simulink model "GFL_hw"  (R2023b)
settings: Solver=FixedStepAuto  StartTime=0.0  StopTime=Inf  RelTol=1e-3  EnableMultiTasking=on
values from neighbouring files (symbols this model uses):
  alpha_c = 2*pi*400    (= 2513.27412287)    [init_hw.m]    (also in init_psc_hw.m)
  L_f = 1e-3    (= 0.001)    [init_hw.m]    (also in init_psc_hw.m)
  T_pwm = f_clk/(div*f_sw*carr)    (= 9000)    [init_hw.m]    (also in init_psc_hw.m)
  T_s = 1/(2*f_sw)    (= 0.0001)    [init_hw.m]    (also in init_psc_hw.m)
  u_gN = 24    [init_hw.m]    (also in init_psc_hw.m)
  w0_pll = 2*pi*20    (= 125.663706144)    [init_hw.m]    (also in init_psc_hw.m)
undefined symbols (not defined in the file or in its folder): Down, GPTRIP1SEL, GPTRIP2SEL, TZ1, TZ2, Up, w_g
libraries: c2802xlib x14, c2806xlib x5
settings Model: SimulationMode=external  ExtModeTrigDuration=15  Creator=maatt  LastModifiedBy=maatt
settings OptimizationCC: DefaultUnderspecifiedDataType=single  EnhancedBackFolding=on  PassReuseOutputArgsAs=Individual arguments  MaxStackSize=1024  OptimizeBlockOrder=speed  DifferentSizesBufferReuse=on  OptimizationCustomize=off  EfficientTunableParamExpr=on
settings DebuggingCC: ParameterTunabilityLossMsg=error
settings HardwareCC: ProdBitPerChar=16  ProdBitPerInt=16  ProdBitPerPointer=32  ProdBitPerSizeT=32  ProdBitPerPtrDiffT=32  ProdLargestAtomicInteger=Integer  ProdLargestAtomicFloat=None  ProdWordSize=16  ProdLongLongMode=on  ProdHWDeviceType=Texas Instruments->C2000  HardwareBoardFeatureSet=SoCBlockset
settings ModelReferenceCC: ModelReferenceNumInstancesAllowed=Single
settings SFSimCC: MATLABDynamicMemAlloc=off
settings RTWCC: Description=Embedded Coder  SystemTargetFile=ert.tlc  HardwareBoard=TI Piccolo F28069M LaunchPad  TemplateMakefile=ert_default_tmf  Toolchain=Texas Instruments Code Composer Studio (C2000)  CodeProfilingSaveOptions=MetricsOnly
settings CodeAppCC: ForceParamTrailComments=on  IgnoreCustomStorageClasses=off  OperatorAnnotations=on  SimulinkDataObjDesc=on  SFDataObjDesc=on  InsertBlockDesc=on
settings ERTTargetCC: CodeReplacementLibrary=TI C28x  ExtModeTransport=4  ExtModeStaticAlloc=on  ExtModeAutomaticAllocSize=off  ExtModeStaticAllocSize=2000  ExtModeMexFile=ext_xcp  ExtModeIntrfLevel=Level2 - Open

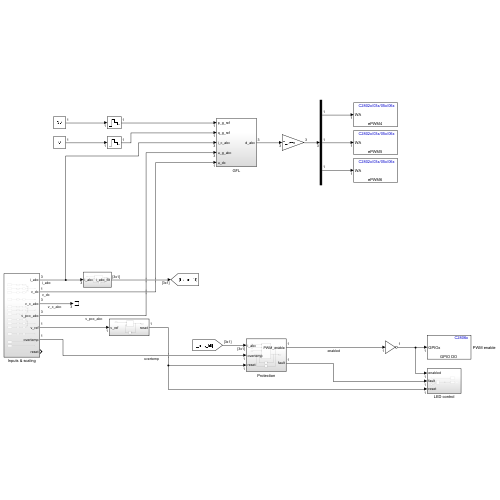
[thumbnail: Simulink's stored preview of the top-level diagram]
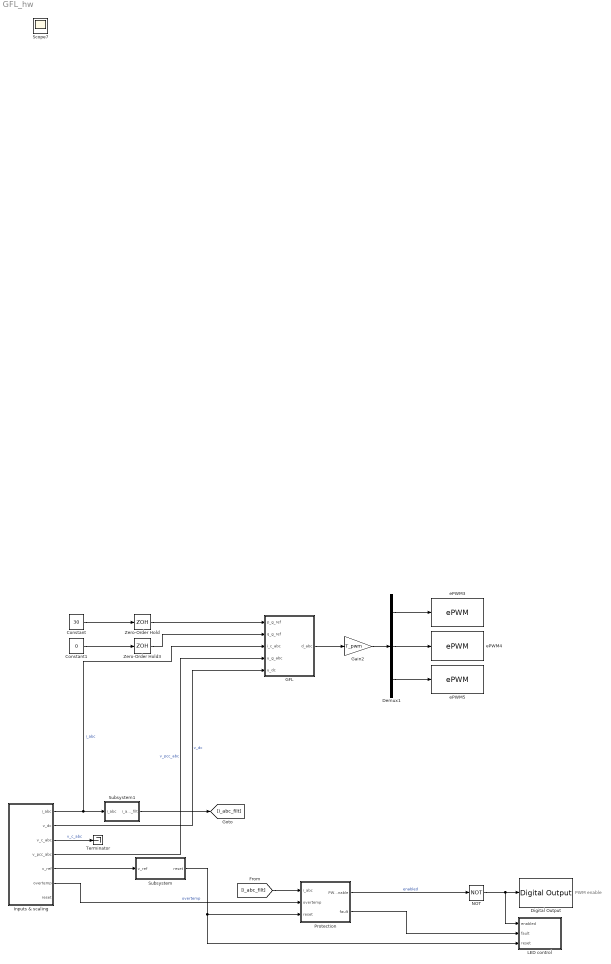
== system GFL_hw ==
  note: PWM enable
  Constant : Constant  Value=30  SampleTime=T_s
  Constant1 : Constant  Value=0  SampleTime=T_s
  Demux1 : Demux  Outputs=3
  Digital Output : c2806xlib/Digital Output  GPIO_Number=GPIO50~GPIO55  GPIO_Bit0=off  GPIO_BIT0_Toggle=off  GPIO_Bit1=off  GPIO_BIT1_Toggle=off  GPIO_Bit2=off  GPIO_BIT2_Toggle=off  GPIO_Bit3=off  GPIO_BIT3_Toggle=off  GPIO_Bit4=on  GPIO_BIT4_Toggle=off  GPIO_Bit5=off  GPIO_BIT5_Toggle=off  GPIO_Bit6=off  GPIO_BIT6_Toggle=off  GPIO_Bit7=off  GPIO_BIT7_Toggle=off
  GFL : Subsystem
  Gain2 : Gain  Gain=T_pwm
  Inputs & scaling : Subsystem
  LED control : Subsystem
  NOT : Logic  Operator=NOT  IconShape=distinctive  AllPortsSameDT=off  OutDataTypeStr=boolean
  Protection : Subsystem
  Subsystem : Subsystem
  Subsystem1 : Subsystem
  Terminator : Terminator
  Zero-Order Hold : ZeroOrderHold  SampleTime=T_s
  Zero-Order Hold3 : ZeroOrderHold  SampleTime=T_s
  ePWM3 : c2802xlib/ePWM  PwmType=C2000  useModule=ePWM4  ePWMxLINKTBPRD=Not Linked  periodUnits=Clock cycles  timerSource=Specify via dialog  timerPeriod_clk=T_pwm + 1  timerPeriod_sec=0.0001  tbshadow=Counter equals to zero  countingMode=Up-Down  phaseActiveEnable=Disable  phaseDirection=Count down after sync  phaseActive=0  synchronizationEnable=off  dcaevt1Sync=off  dcbevt1Sync=off  synchronizationOption=Counter equals to zero (CTR=Zero)  dcbevt1SyncOut=off  dcaevt1SyncOut=off  cmpdSyncOut=off  cmpcSyncOut=off  cmpbSyncOut=off  zeroSyncOut=off  swfSyncOut=off  perSynchronizationOption=Counter equals to period (CTR=PRD)  clockPrescale=1  HSclockPrescale=1  enswap=off  ePWMxAStatus=on  ePWMxAactionLogic1=Do nothing  ePWMxAactionLogic2=Do nothing  ePWMxAactionLogic3=Clear  ePWMxAactionLogic4=Set  ePWMxAactionLogic5=Do nothing  ePWMxAactionLogic6=Do nothing  ePWMxACSFenable=off  ePWMxACSFvalue=Forcing disable  ePWMxASFreload=Zero  ePWMxBStatus=off  ePWMxBactionLogic1=Set  ePWMxBactionLogic2=Clear  ePWMxBactionLogic3=Do nothing  ePWMxBactionLogic4=Do nothing  ePWMxBactionLogic5=Clear  ePWMxBactionLogic6=Set  ePWMxBCSFenable=off  ePWMxBCSFvalue=Forcing disable  ePWMxBSFreload=Zero  ePWNxBOutWay=on  ePWMxLINKCMPA=Not Linked  CMPAUnits=Clock cycles  CMPASource=Input port  CMPAValue_per=50  CMPAValue_clk=T_pwm/2  enCMPAshadow=Counter equals to zero (CTR=Zero)  ePWMxLINKCMPB=Not Linked  CMPBUnits=Clock cycles  CMPBSource=Specify via dialog  CMPBValue_per=50  CMPBValue_clk=T_pwm/2  enCMPBshadow=Counter equals to zero (CTR=Zero)  ePWMxLINKCMPC=Not Linked  CMPCUnits=Clock cycles  CMPCSource=Specify via dialog  CMPCValue_per=50  CMPCValue_clk=32000  enCMPCshadow=Counter equals to zero (CTR=Zero)  ePWMxLINKCMPD=Not Linked  CMPDUnits=Clock cycles  CMPDSource=Specify via dialog  CMPDValue_per=50  CMPDValue_clk=32000  enCMPDshadow=Counter equals to zero (CTR=Zero)  enableDBePWMxA=on  enableDBePWMxB=on  enhalfcycle=off  DBpolarity=Active high complementary (AHC)  DBedgeDelay=Positive  DBSource_ePWMxA=ePWMxA  DBSource_ePWMxB=ePWMxA  DBPeriodUnits=Clock cycles  DBperiodSource=Specify via dialog  REDperiod=15  FEDperiod=15  REDperiod_sec=0  FEDperiod_sec=0  LoadModeDBRED=Immediate without using shadow  LoadModeDBFED=Immediate without using shadow  adcstartModuleA=off  adcrequestEventA=First event  adcstartEventA=Counter equals to zero (CTR=Zero)  adcstartEventA_type2=Digital Compare Module A Event 1 start of conversion (DCAEVT1.soc)  adcstartModuleB=off  adcrequestEventB=First event  adcstartEventB=Counter equals to zero (CTR=Zero)  adcstartEventB_type2=Counter equals to zero (CTR=Zero)  intEn=off  intPrd=First event  intSel=Counter equals to zero (CTR=Zero)  intSel_type2=Counter equals to zero (CTR=Zero)  hrpe=off  enHRPWM=off  HRPWM_LoadMode=Counter equals to period (CTR=PRD)  HRPWM_CTLMode=Duty or Period control mode  HRPWM_EDGMode=Both edge  hrpeb=off  enHRPWMB=off  HRPWM_LoadModeB=Counter equals to zero (CTR=ZERO)  HRPWM_CTLModeB=Duty or Period control mode  HRPWM_EDGModeB=Both edge  enHRDBRED=off  enHRDBFED=off  enSFO=on  enautoconv=on  chopperEnable=off  chopperFrequency=1  chopperFirstwidth=1  chopperDuty=12.5%  tripZonesource=Specify via dialog  tzselOSHT1=off  tzselOSHT2=off  tzselOSHT3=off  tzselOSHDCAEV1=off  tzselOSHDCBEV1=off  tzselCBC1=off  tzselCBC2=off  tzselCBC3=off  tzselCBCDCAEV2=off  tzselCBCDCBEV2=off  tzselOSHT4=off  tzselOSHT5=off  tzselOSHT6=off  tzselCBC4=off  tzselCBC5=off  tzselCBC6=off  enTzOstIntr=off  enTzCbcIntr=off  enTzDCAEVT1Intr=off  enTzDCAEVT2Intr=off  enTzDCBEVT1Intr=off  enTzDCBEVT2Intr=off  ePWMxAforced=No action  ePWMxBforced=No action  DCAEVT1forced=No action  DCBEVT1forced=No action  DCAEVT2forced=No action  DCBEVT2forced=No action  dcah=Trip Zone 1 input (TZ1)  dcal=Trip Zone 1 input (TZ1)  dcbh=Trip Zone 1 input (TZ1)  dcbl=Trip Zone 1 input (TZ1)  dcah_type2=GPTRIP1SEL/(TZ1)  dcal_type2=GPTRIP2SEL/(TZ2)  dcbh_type2=GPTRIP1SEL/(TZ1)  dcbl_type2=GPTRIP2SEL/(TZ2)  gendcaevt1=Event disabled  gendcaevt2=Event disabled  gendcbevt1=Event disabled  gendcbevt2=Event disabled  dcaevt1src=DCAEVT1 with sync  dcaevt2src=DCAEVT2 with sync  dcbevt1src=DCBEVT1 with sync  dcbevt2src=DCBEVT2 with sync  pulsesel=Counter equals to zero (CTR=Zero)  blankinv=off  blankoffset=0  blankwidth=0  evsrcsel=Filtered version of DCAEVT1 (DCAEVT1FILT)  encape=off
      settings: LibrarySourceBlock=c2806xlib/ePWM
  ePWM4 : c2802xlib/ePWM  PwmType=C2000  useModule=ePWM5  ePWMxLINKTBPRD=Not Linked  periodUnits=Clock cycles  timerSource=Specify via dialog  timerPeriod_clk=T_pwm + 1  timerPeriod_sec=0.0001  tbshadow=Counter equals to zero  countingMode=Up-Down  phaseActiveEnable=Disable  phaseDirection=Count down after sync  phaseActive=0  synchronizationEnable=off  dcaevt1Sync=off  dcbevt1Sync=off  synchronizationOption=Counter equals to zero (CTR=Zero)  dcbevt1SyncOut=off  dcaevt1SyncOut=off  cmpdSyncOut=off  cmpcSyncOut=off  cmpbSyncOut=off  zeroSyncOut=off  swfSyncOut=off  perSynchronizationOption=Counter equals to period (CTR=PRD)  clockPrescale=1  HSclockPrescale=1  enswap=off  ePWMxAStatus=on  ePWMxAactionLogic1=Do nothing  ePWMxAactionLogic2=Do nothing  ePWMxAactionLogic3=Clear  ePWMxAactionLogic4=Set  ePWMxAactionLogic5=Do nothing  ePWMxAactionLogic6=Do nothing  ePWMxACSFenable=off  ePWMxACSFvalue=Forcing disable  ePWMxASFreload=Zero  ePWMxBStatus=off  ePWMxBactionLogic1=Set  ePWMxBactionLogic2=Clear  ePWMxBactionLogic3=Do nothing  ePWMxBactionLogic4=Do nothing  ePWMxBactionLogic5=Clear  ePWMxBactionLogic6=Set  ePWMxBCSFenable=off  ePWMxBCSFvalue=Forcing disable  ePWMxBSFreload=Zero  ePWNxBOutWay=on  ePWMxLINKCMPA=Not Linked  CMPAUnits=Clock cycles  CMPASource=Input port  CMPAValue_per=50  CMPAValue_clk=T_pwm/2  enCMPAshadow=Counter equals to zero (CTR=Zero)  ePWMxLINKCMPB=Not Linked  CMPBUnits=Clock cycles  CMPBSource=Specify via dialog  CMPBValue_per=50  CMPBValue_clk=T_pwm/2  enCMPBshadow=Counter equals to zero (CTR=Zero)  ePWMxLINKCMPC=Not Linked  CMPCUnits=Clock cycles  CMPCSource=Specify via dialog  CMPCValue_per=50  CMPCValue_clk=32000  enCMPCshadow=Counter equals to zero (CTR=Zero)  ePWMxLINKCMPD=Not Linked  CMPDUnits=Clock cycles  CMPDSource=Specify via dialog  CMPDValue_per=50  CMPDValue_clk=32000  enCMPDshadow=Counter equals to zero (CTR=Zero)  enableDBePWMxA=on  enableDBePWMxB=on  enhalfcycle=off  DBpolarity=Active high complementary (AHC)  DBedgeDelay=Positive  DBSource_ePWMxA=ePWMxA  DBSource_ePWMxB=ePWMxA  DBPeriodUnits=Clock cycles  DBperiodSource=Specify via dialog  REDperiod=15  FEDperiod=15  REDperiod_sec=0  FEDperiod_sec=0  LoadModeDBRED=Immediate without using shadow  LoadModeDBFED=Immediate without using shadow  adcstartModuleA=off  adcrequestEventA=First event  adcstartEventA=Counter equals to zero (CTR=Zero)  adcstartEventA_type2=Digital Compare Module A Event 1 start of conversion (DCAEVT1.soc)  adcstartModuleB=off  adcrequestEventB=First event  adcstartEventB=Counter equals to zero (CTR=Zero)  adcstartEventB_type2=Counter equals to zero (CTR=Zero)  intEn=off  intPrd=First event  intSel=Counter equals to zero (CTR=Zero)  intSel_type2=Counter equals to zero (CTR=Zero)  hrpe=off  enHRPWM=off  HRPWM_LoadMode=Counter equals to period (CTR=PRD)  HRPWM_CTLMode=Duty or Period control mode  HRPWM_EDGMode=Both edge  hrpeb=off  enHRPWMB=off  HRPWM_LoadModeB=Counter equals to zero (CTR=ZERO)  HRPWM_CTLModeB=Duty or Period control mode  HRPWM_EDGModeB=Both edge  enHRDBRED=off  enHRDBFED=off  enSFO=on  enautoconv=on  chopperEnable=off  chopperFrequency=1  chopperFirstwidth=1  chopperDuty=12.5%  tripZonesource=Specify via dialog  tzselOSHT1=off  tzselOSHT2=off  tzselOSHT3=off  tzselOSHDCAEV1=off  tzselOSHDCBEV1=off  tzselCBC1=off  tzselCBC2=off  tzselCBC3=off  tzselCBCDCAEV2=off  tzselCBCDCBEV2=off  tzselOSHT4=off  tzselOSHT5=off  tzselOSHT6=off  tzselCBC4=off  tzselCBC5=off  tzselCBC6=off  enTzOstIntr=off  enTzCbcIntr=off  enTzDCAEVT1Intr=off  enTzDCAEVT2Intr=off  enTzDCBEVT1Intr=off  enTzDCBEVT2Intr=off  ePWMxAforced=No action  ePWMxBforced=No action  DCAEVT1forced=No action  DCBEVT1forced=No action  DCAEVT2forced=No action  DCBEVT2forced=No action  dcah=Trip Zone 1 input (TZ1)  dcal=Trip Zone 1 input (TZ1)  dcbh=Trip Zone 1 input (TZ1)  dcbl=Trip Zone 1 input (TZ1)  dcah_type2=GPTRIP1SEL/(TZ1)  dcal_type2=GPTRIP2SEL/(TZ2)  dcbh_type2=GPTRIP1SEL/(TZ1)  dcbl_type2=GPTRIP2SEL/(TZ2)  gendcaevt1=Event disabled  gendcaevt2=Event disabled  gendcbevt1=Event disabled  gendcbevt2=Event disabled  dcaevt1src=DCAEVT1 with sync  dcaevt2src=DCAEVT2 with sync  dcbevt1src=DCBEVT1 with sync  dcbevt2src=DCBEVT2 with sync  pulsesel=Counter equals to zero (CTR=Zero)  blankinv=off  blankoffset=0  blankwidth=0  evsrcsel=Filtered version of DCAEVT1 (DCAEVT1FILT)  encape=off
      settings: LibrarySourceBlock=c2806xlib/ePWM
  ePWM5 : c2802xlib/ePWM  PwmType=C2000  useModule=ePWM6  ePWMxLINKTBPRD=Not Linked  periodUnits=Clock cycles  timerSource=Specify via dialog  timerPeriod_clk=T_pwm + 1  timerPeriod_sec=0.0001  tbshadow=Counter equals to zero  countingMode=Up-Down  phaseActiveEnable=Disable  phaseDirection=Count down after sync  phaseActive=0  synchronizationEnable=off  dcaevt1Sync=off  dcbevt1Sync=off  synchronizationOption=Counter equals to zero (CTR=Zero)  dcbevt1SyncOut=off  dcaevt1SyncOut=off  cmpdSyncOut=off  cmpcSyncOut=off  cmpbSyncOut=off  zeroSyncOut=off  swfSyncOut=off  perSynchronizationOption=Counter equals to period (CTR=PRD)  clockPrescale=1  HSclockPrescale=1  enswap=off  ePWMxAStatus=on  ePWMxAactionLogic1=Do nothing  ePWMxAactionLogic2=Do nothing  ePWMxAactionLogic3=Clear  ePWMxAactionLogic4=Set  ePWMxAactionLogic5=Do nothing  ePWMxAactionLogic6=Do nothing  ePWMxACSFenable=off  ePWMxACSFvalue=Forcing disable  ePWMxASFreload=Zero  ePWMxBStatus=off  ePWMxBactionLogic1=Set  ePWMxBactionLogic2=Clear  ePWMxBactionLogic3=Do nothing  ePWMxBactionLogic4=Do nothing  ePWMxBactionLogic5=Clear  ePWMxBactionLogic6=Set  ePWMxBCSFenable=off  ePWMxBCSFvalue=Forcing disable  ePWMxBSFreload=Zero  ePWNxBOutWay=on  ePWMxLINKCMPA=Not Linked  CMPAUnits=Clock cycles  CMPASource=Input port  CMPAValue_per=50  CMPAValue_clk=T_pwm/2  enCMPAshadow=Counter equals to zero (CTR=Zero)  ePWMxLINKCMPB=Not Linked  CMPBUnits=Clock cycles  CMPBSource=Specify via dialog  CMPBValue_per=50  CMPBValue_clk=T_pwm/2  enCMPBshadow=Counter equals to zero (CTR=Zero)  ePWMxLINKCMPC=Not Linked  CMPCUnits=Clock cycles  CMPCSource=Specify via dialog  CMPCValue_per=50  CMPCValue_clk=32000  enCMPCshadow=Counter equals to zero (CTR=Zero)  ePWMxLINKCMPD=Not Linked  CMPDUnits=Clock cycles  CMPDSource=Specify via dialog  CMPDValue_per=50  CMPDValue_clk=32000  enCMPDshadow=Counter equals to zero (CTR=Zero)  enableDBePWMxA=on  enableDBePWMxB=on  enhalfcycle=off  DBpolarity=Active high complementary (AHC)  DBedgeDelay=Positive  DBSource_ePWMxA=ePWMxA  DBSource_ePWMxB=ePWMxA  DBPeriodUnits=Clock cycles  DBperiodSource=Specify via dialog  REDperiod=15  FEDperiod=15  REDperiod_sec=0  FEDperiod_sec=0  LoadModeDBRED=Immediate without using shadow  LoadModeDBFED=Immediate without using shadow  adcstartModuleA=off  adcrequestEventA=First event  adcstartEventA=Counter equals to zero (CTR=Zero)  adcstartEventA_type2=Digital Compare Module A Event 1 start of conversion (DCAEVT1.soc)  adcstartModuleB=off  adcrequestEventB=First event  adcstartEventB=Counter equals to zero (CTR=Zero)  adcstartEventB_type2=Counter equals to zero (CTR=Zero)  intEn=off  intPrd=First event  intSel=Counter equals to zero (CTR=Zero)  intSel_type2=Counter equals to zero (CTR=Zero)  hrpe=off  enHRPWM=off  HRPWM_LoadMode=Counter equals to period (CTR=PRD)  HRPWM_CTLMode=Duty or Period control mode  HRPWM_EDGMode=Both edge  hrpeb=off  enHRPWMB=off  HRPWM_LoadModeB=Counter equals to zero (CTR=ZERO)  HRPWM_CTLModeB=Duty or Period control mode  HRPWM_EDGModeB=Both edge  enHRDBRED=off  enHRDBFED=off  enSFO=on  enautoconv=on  chopperEnable=off  chopperFrequency=1  chopperFirstwidth=1  chopperDuty=12.5%  tripZonesource=Specify via dialog  tzselOSHT1=off  tzselOSHT2=off  tzselOSHT3=off  tzselOSHDCAEV1=off  tzselOSHDCBEV1=off  tzselCBC1=off  tzselCBC2=off  tzselCBC3=off  tzselCBCDCAEV2=off  tzselCBCDCBEV2=off  tzselOSHT4=off  tzselOSHT5=off  tzselOSHT6=off  tzselCBC4=off  tzselCBC5=off  tzselCBC6=off  enTzOstIntr=off  enTzCbcIntr=off  enTzDCAEVT1Intr=off  enTzDCAEVT2Intr=off  enTzDCBEVT1Intr=off  enTzDCBEVT2Intr=off  ePWMxAforced=No action  ePWMxBforced=No action  DCAEVT1forced=No action  DCBEVT1forced=No action  DCAEVT2forced=No action  DCBEVT2forced=No action  dcah=Trip Zone 1 input (TZ1)  dcal=Trip Zone 1 input (TZ1)  dcbh=Trip Zone 1 input (TZ1)  dcbl=Trip Zone 1 input (TZ1)  dcah_type2=GPTRIP1SEL/(TZ1)  dcal_type2=GPTRIP2SEL/(TZ2)  dcbh_type2=GPTRIP1SEL/(TZ1)  dcbl_type2=GPTRIP2SEL/(TZ2)  gendcaevt1=Event disabled  gendcaevt2=Event disabled  gendcbevt1=Event disabled  gendcbevt2=Event disabled  dcaevt1src=DCAEVT1 with sync  dcaevt2src=DCAEVT2 with sync  dcbevt1src=DCBEVT1 with sync  dcbevt2src=DCBEVT2 with sync  pulsesel=Counter equals to zero (CTR=Zero)  blankinv=off  blankoffset=0  blankwidth=0  evsrcsel=Filtered version of DCAEVT1 (DCAEVT1FILT)  encape=off
      settings: LibrarySourceBlock=c2806xlib/ePWM
  Scope7 : Scope
  wires:
  Demux1/1 -> ePWM3/1
  Demux1/2 -> ePWM4/1
  Gain2/1 -> Demux1/1
  Demux1/3 -> ePWM5/1
  [i_abc_filt] -> Protection/1(i_abc)
  Protection/1(PWM_enable) -> NOT/1  "enabled"
  Protection/2(fault) -> LED control/2(fault)
  Inputs & scaling/6(overtemp) -> Protection/2(overtemp)  "overtemp"
  Inputs & scaling/1(i_abc) -> GFL/3(i_c_abc), Subsystem1/1(i_abc)  "i_abc"
  Inputs & scaling/5(v_ref) -> Subsystem/1(v_ref)
  Inputs & scaling/3(v_c_abc) -> Terminator/1  "v_c_abc"
  Inputs & scaling/4(v_pcc_abc) -> GFL/4(u_g_abc)  "v_pcc_abc"
  NOT/1 -> LED control/1(enabled), Digital Output/1
  Subsystem/1(reset) -> Protection/3(reset), LED control/3(reset)
  Subsystem1/1(i_abc_filt) -> [i_abc_filt]
  GFL/1(d_abc) -> Gain2/1
  Zero-Order Hold/1 -> GFL/1(p_g_ref)
  Constant1/1 -> Zero-Order Hold3/1
  Zero-Order Hold3/1 -> GFL/2(q_g_ref)
  Inputs & scaling/2(v_dc) -> GFL/5(u_dc)  "v_dc"
  Constant/1 -> Zero-Order Hold/1

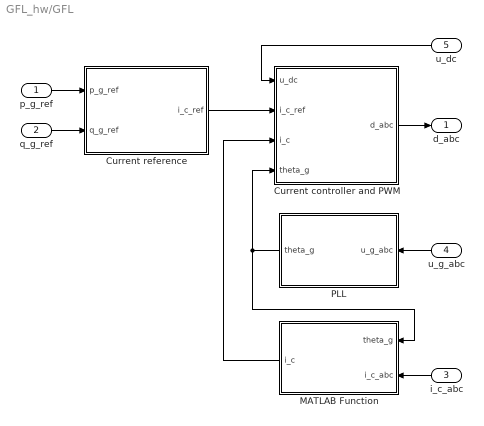
== system GFL_hw/GFL ==
  p_g_ref : Inport
  q_g_ref : Inport  Port=2
  i_c_abc : Inport  Port=3
  u_g_abc : Inport  Port=4
  u_dc : Inport  Port=5
  Current controller and PWM : Subsystem
  Current reference : MATLAB Function  TreatAsAtomicUnit=on
  MATLAB Function : MATLAB Function  TreatAsAtomicUnit=on
  PLL : Subsystem
  d_abc : Outport
  wires:
  i_c_abc/1 -> MATLAB Function/2(i_c_abc)
  Current controller and PWM/1(d_abc) -> d_abc/1
  Current reference/1(i_c_ref) -> Current controller and PWM/2(i_c_ref)
  MATLAB Function/1(i_c) -> Current controller and PWM/3(i_c)
  q_g_ref/1 -> Current reference/2(q_g_ref)
  p_g_ref/1 -> Current reference/1(p_g_ref)
  u_g_abc/1 -> PLL/1(u_g_abc)
  PLL/1(theta_g) -> MATLAB Function/1(theta_g), Current controller and PWM/4(theta_g)
  u_dc/1 -> Current controller and PWM/1(u_dc)

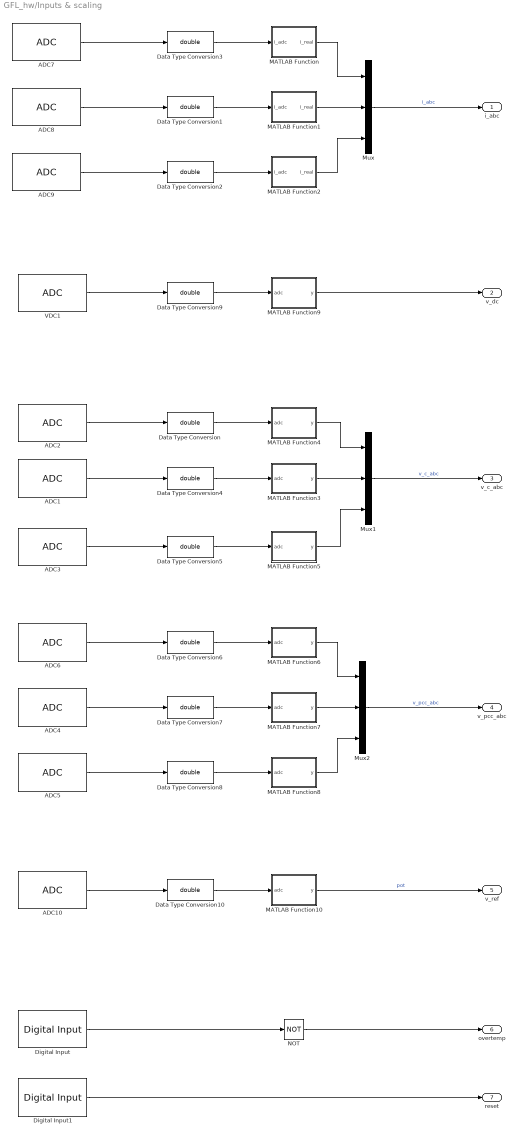
== system GFL_hw/Inputs & scaling ==
  ADC1 : c2802xlib/ADC  blkParamProc=C2000  ADCModule=1  samplingMode=Single sample mode  ADCResolution=12-bit (Single-ended input)  useSOC1=SOC5  useSOC2=SOC0_SOC1  SOCAcquisitionWindow=15  SOCTriggerSource=Software  SOCInterruptTrigger=No ADCINT  Ts=T_s  dType=uint16  postInterrupt=off  interruptSel=ADCINT1  ADCINTContinuous=off  endma=off  chdma=1  conv1=ADCINA5  conv2=ADCINA0 and ADCINB0  conv1_Type4=ADCIN0  conv2_Type4=ADCIN0 and ADCIN1
      settings: LibrarySourceBlock=c2806xlib/ADC
  ADC10 : c2802xlib/ADC  blkParamProc=C2000  ADCModule=1  samplingMode=Single sample mode  ADCResolution=12-bit (Single-ended input)  useSOC1=SOC10  useSOC2=SOC0_SOC1  SOCAcquisitionWindow=15  SOCTriggerSource=Software  SOCInterruptTrigger=No ADCINT  Ts=T_s  dType=uint16  postInterrupt=off  interruptSel=ADCINT1  ADCINTContinuous=off  endma=off  chdma=1  conv1=ADCINB2  conv2=ADCINA0 and ADCINB0  conv1_Type4=ADCIN0  conv2_Type4=ADCIN0 and ADCIN1
      settings: LibrarySourceBlock=c2806xlib/ADC
  ADC2 : c2802xlib/ADC  blkParamProc=C2000  ADCModule=1  samplingMode=Single sample mode  ADCResolution=12-bit (Single-ended input)  useSOC1=SOC4  useSOC2=SOC0_SOC1  SOCAcquisitionWindow=15  SOCTriggerSource=Software  SOCInterruptTrigger=No ADCINT  Ts=T_s  dType=uint16  postInterrupt=off  interruptSel=ADCINT1  ADCINTContinuous=off  endma=off  chdma=1  conv1=ADCINB4  conv2=ADCINA0 and ADCINB0  conv1_Type4=ADCIN0  conv2_Type4=ADCIN0 and ADCIN1
      settings: LibrarySourceBlock=c2806xlib/ADC
  ADC3 : c2802xlib/ADC  blkParamProc=C2000  ADCModule=1  samplingMode=Single sample mode  ADCResolution=12-bit (Single-ended input)  useSOC1=SOC6  useSOC2=SOC0_SOC1  SOCAcquisitionWindow=15  SOCTriggerSource=Software  SOCInterruptTrigger=No ADCINT  Ts=T_s  dType=uint16  postInterrupt=off  interruptSel=ADCINT1  ADCINTContinuous=off  endma=off  chdma=1  conv1=ADCINB5  conv2=ADCINA0 and ADCINB0  conv1_Type4=ADCIN0  conv2_Type4=ADCIN0 and ADCIN1
      settings: LibrarySourceBlock=c2806xlib/ADC
  ADC4 : c2802xlib/ADC  blkParamProc=C2000  ADCModule=1  samplingMode=Single sample mode  ADCResolution=12-bit (Single-ended input)  useSOC1=SOC8  useSOC2=SOC0_SOC1  SOCAcquisitionWindow=15  SOCTriggerSource=Software  SOCInterruptTrigger=No ADCINT  Ts=T_s  dType=uint16  postInterrupt=off  interruptSel=ADCINT1  ADCINTContinuous=off  endma=off  chdma=1  conv1=ADCINB1  conv2=ADCINA0 and ADCINB0  conv1_Type4=ADCIN0  conv2_Type4=ADCIN0 and ADCIN1
      settings: LibrarySourceBlock=c2806xlib/ADC
  ADC5 : c2802xlib/ADC  blkParamProc=C2000  ADCModule=1  samplingMode=Single sample mode  ADCResolution=12-bit (Single-ended input)  useSOC1=SOC9  useSOC2=SOC0_SOC1  SOCAcquisitionWindow=15  SOCTriggerSource=Software  SOCInterruptTrigger=No ADCINT  Ts=T_s  dType=uint16  postInterrupt=off  interruptSel=ADCINT1  ADCINTContinuous=off  endma=off  chdma=1  conv1=ADCINA2  conv2=ADCINA0 and ADCINB0  conv1_Type4=ADCIN0  conv2_Type4=ADCIN0 and ADCIN1
      settings: LibrarySourceBlock=c2806xlib/ADC
  ADC6 : c2802xlib/ADC  blkParamProc=C2000  ADCModule=1  samplingMode=Single sample mode  ADCResolution=12-bit (Single-ended input)  useSOC1=SOC7  useSOC2=SOC0_SOC1  SOCAcquisitionWindow=15  SOCTriggerSource=Software  SOCInterruptTrigger=No ADCINT  Ts=T_s  dType=uint16  postInterrupt=off  interruptSel=ADCINT1  ADCINTContinuous=off  endma=off  chdma=1  conv1=ADCINA7  conv2=ADCINA0 and ADCINB0  conv1_Type4=ADCIN0  conv2_Type4=ADCIN0 and ADCIN1
      settings: LibrarySourceBlock=c2806xlib/ADC
  ADC7 : c2802xlib/ADC  blkParamProc=C2000  ADCModule=1  samplingMode=Single sample mode  ADCResolution=12-bit (Single-ended input)  useSOC1=SOC0  useSOC2=SOC0_SOC1  SOCAcquisitionWindow=15  SOCTriggerSource=Software  SOCInterruptTrigger=No ADCINT  Ts=T_s  dType=uint16  postInterrupt=off  interruptSel=ADCINT1  ADCINTContinuous=off  endma=off  chdma=1  conv1=ADCINA3  conv2=ADCINA0 and ADCINB0  conv1_Type4=ADCIN0  conv2_Type4=ADCIN0 and ADCIN1
      settings: LibrarySourceBlock=c2806xlib/ADC
  ADC8 : c2802xlib/ADC  blkParamProc=C2000  ADCModule=1  samplingMode=Single sample mode  ADCResolution=12-bit (Single-ended input)  useSOC1=SOC1  useSOC2=SOC0_SOC1  SOCAcquisitionWindow=15  SOCTriggerSource=Software  SOCInterruptTrigger=No ADCINT  Ts=T_s  dType=uint16  postInterrupt=on  interruptSel=ADCINT1  ADCINTContinuous=off  endma=off  chdma=1  conv1=ADCINB3  conv2=ADCINA0 and ADCINB0  conv1_Type4=ADCIN0  conv2_Type4=ADCIN0 and ADCIN1
      settings: LibrarySourceBlock=c2806xlib/ADC
  ADC9 : c2802xlib/ADC  blkParamProc=C2000  ADCModule=1  samplingMode=Single sample mode  ADCResolution=12-bit (Single-ended input)  useSOC1=SOC2  useSOC2=SOC0_SOC1  SOCAcquisitionWindow=15  SOCTriggerSource=Software  SOCInterruptTrigger=No ADCINT  Ts=T_s  dType=uint16  postInterrupt=off  interruptSel=ADCINT1  ADCINTContinuous=off  endma=off  chdma=1  conv1=ADCINA4  conv2=ADCINA0 and ADCINB0  conv1_Type4=ADCIN0  conv2_Type4=ADCIN0 and ADCIN1
      settings: LibrarySourceBlock=c2806xlib/ADC
  Data Type Conversion{,1..10} (11 alike) : DataTypeConversion  OutDataTypeStr=double  SaturateOnIntegerOverflow=off  RndMeth=Floor
  Digital Input : c2806xlib/Digital Input  GPIO_Number=GPIO8~GPIO15  GPIO_Bit0=off  GPIO_Bit1=off  GPIO_Bit2=off  GPIO_Bit3=off  GPIO_Bit4=off  GPIO_Bit5=on  GPIO_Bit6=off  GPIO_Bit7=off  sampleTime=T_s  dataType=boolean  GPIO_Bit0_Qualification=Sync to SYSCLKOUT  GPIO_Bit1_Qualification=Sync to SYSCLKOUT  GPIO_Bit2_Qualification=Sync to SYSCLKOUT  GPIO_Bit3_Qualification=Sync to SYSCLKOUT  GPIO_Bit4_Qualification=Sync to SYSCLKOUT  GPIO_Bit5_Qualification=Sync to SYSCLKOUT  GPIO_Bit6_Qualification=Sync to SYSCLKOUT  GPIO_Bit7_Qualification=Sync to SYSCLKOUT  Qualification_Period=-1
  Digital Input1 : c2806xlib/Digital Input  GPIO_Number=GPIO0~GPIO7  GPIO_Bit0=off  GPIO_Bit1=off  GPIO_Bit2=off  GPIO_Bit3=off  GPIO_Bit4=off  GPIO_Bit5=on  GPIO_Bit6=off  GPIO_Bit7=off  sampleTime=T_s  dataType=boolean  GPIO_Bit0_Qualification=Sync to SYSCLKOUT  GPIO_Bit1_Qualification=Sync to SYSCLKOUT  GPIO_Bit2_Qualification=Sync to SYSCLKOUT  GPIO_Bit3_Qualification=Sync to SYSCLKOUT  GPIO_Bit4_Qualification=Sync to SYSCLKOUT  GPIO_Bit5_Qualification=Sync to SYSCLKOUT  GPIO_Bit6_Qualification=Sync to SYSCLKOUT  GPIO_Bit7_Qualification=Sync to SYSCLKOUT  Qualification_Period=-1
  MATLAB Function : MATLAB Function  TreatAsAtomicUnit=on
  MATLAB Function1 : MATLAB Function  TreatAsAtomicUnit=on
  MATLAB Function10 : MATLAB Function  TreatAsAtomicUnit=on
  MATLAB Function2 : MATLAB Function  TreatAsAtomicUnit=on
  MATLAB Function3 : MATLAB Function  TreatAsAtomicUnit=on
  MATLAB Function4 : MATLAB Function  TreatAsAtomicUnit=on
  MATLAB Function5 : MATLAB Function  TreatAsAtomicUnit=on
  MATLAB Function6 : MATLAB Function  TreatAsAtomicUnit=on
  MATLAB Function7 : MATLAB Function  TreatAsAtomicUnit=on
  MATLAB Function8 : MATLAB Function  TreatAsAtomicUnit=on
  MATLAB Function9 : MATLAB Function  TreatAsAtomicUnit=on
  Mux : Mux  Inputs=3
  Mux1 : Mux  Inputs=3
  Mux2 : Mux  Inputs=3
  NOT : Logic  Operator=NOT  IconShape=distinctive  AllPortsSameDT=off  OutDataTypeStr=boolean
  VDC1 : c2802xlib/ADC  blkParamProc=C2000  ADCModule=1  samplingMode=Single sample mode  ADCResolution=12-bit (Single-ended input)  useSOC1=SOC3  useSOC2=SOC0_SOC1  SOCAcquisitionWindow=15  SOCTriggerSource=Software  SOCInterruptTrigger=No ADCINT  Ts=T_s  dType=uint16  postInterrupt=off  interruptSel=ADCINT1  ADCINTContinuous=off  endma=off  chdma=1  conv1=ADCINB7  conv2=ADCINA0 and ADCINB0  conv1_Type4=ADCIN0  conv2_Type4=ADCIN0 and ADCIN1
      settings: LibrarySourceBlock=c2806xlib/ADC
  i_abc : Outport
  v_dc : Outport  Port=2
  v_c_abc : Outport  Port=3
  v_pcc_abc : Outport  Port=4
  v_ref : Outport  Port=5
  overtemp : Outport  Port=6
  reset : Outport  Port=7
  wires:
  MATLAB Function1/1(i_real) -> Mux/2
  ADC9/1 -> Data Type Conversion2/1
  Data Type Conversion3/1 -> MATLAB Function/1(i_adc)
  MATLAB Function/1(i_real) -> Mux/1
  MATLAB Function2/1(i_real) -> Mux/3
  Data Type Conversion1/1 -> MATLAB Function1/1(i_adc)
  ADC7/1 -> Data Type Conversion3/1
  Data Type Conversion2/1 -> MATLAB Function2/1(i_adc)
  ADC8/1 -> Data Type Conversion1/1
  Mux/1 -> i_abc/1  "i_abc"
  Data Type Conversion/1 -> MATLAB Function4/1(adc)
  Data Type Conversion4/1 -> MATLAB Function3/1(adc)
  Data Type Conversion5/1 -> MATLAB Function5/1(adc)
  Data Type Conversion6/1 -> MATLAB Function6/1(adc)
  Data Type Conversion7/1 -> MATLAB Function7/1(adc)
  Data Type Conversion8/1 -> MATLAB Function8/1(adc)
  ADC5/1 -> Data Type Conversion8/1
  ADC4/1 -> Data Type Conversion7/1
  ADC6/1 -> Data Type Conversion6/1
  ADC3/1 -> Data Type Conversion5/1
  ADC1/1 -> Data Type Conversion4/1
  ADC2/1 -> Data Type Conversion/1
  MATLAB Function4/1(y) -> Mux1/1
  MATLAB Function3/1(y) -> Mux1/2
  MATLAB Function5/1(y) -> Mux1/3
  MATLAB Function6/1(y) -> Mux2/1
  MATLAB Function7/1(y) -> Mux2/2
  MATLAB Function8/1(y) -> Mux2/3
  Mux1/1 -> v_c_abc/1  "v_c_abc"
  Mux2/1 -> v_pcc_abc/1  "v_pcc_abc"
  Data Type Conversion9/1 -> MATLAB Function9/1(adc)
  VDC1/1 -> Data Type Conversion9/1
  MATLAB Function9/1(y) -> v_dc/1
  ADC10/1 -> Data Type Conversion10/1
  Data Type Conversion10/1 -> MATLAB Function10/1(adc)
  MATLAB Function10/1(y) -> v_ref/1  "pot"
  NOT/1 -> overtemp/1
  Digital Input/1 -> NOT/1
  Digital Input1/1 -> reset/1

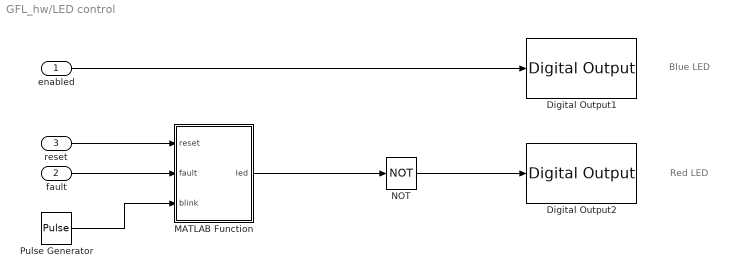
== system GFL_hw/LED control ==
  note: Blue LED
  note: Red LED
  enabled : Inport
  fault : Inport  Port=2
  reset : Inport  Port=3
  Digital Output1 : c2806xlib/Digital Output  GPIO_Number=GPIO32~GPIO39  GPIO_Bit0=off  GPIO_BIT0_Toggle=off  GPIO_Bit1=off  GPIO_BIT1_Toggle=off  GPIO_Bit2=off  GPIO_BIT2_Toggle=off  GPIO_Bit3=off  GPIO_BIT3_Toggle=off  GPIO_Bit4=off  GPIO_BIT4_Toggle=off  GPIO_Bit5=off  GPIO_BIT5_Toggle=off  GPIO_Bit6=off  GPIO_BIT6_Toggle=off  GPIO_Bit7=on  GPIO_BIT7_Toggle=off
  Digital Output2 : c2806xlib/Digital Output  GPIO_Number=GPIO32~GPIO39  GPIO_Bit0=off  GPIO_BIT0_Toggle=off  GPIO_Bit1=off  GPIO_BIT1_Toggle=off  GPIO_Bit2=on  GPIO_BIT2_Toggle=off  GPIO_Bit3=off  GPIO_BIT3_Toggle=off  GPIO_Bit4=off  GPIO_BIT4_Toggle=off  GPIO_Bit5=off  GPIO_BIT5_Toggle=off  GPIO_Bit6=off  GPIO_BIT6_Toggle=off  GPIO_Bit7=off  GPIO_BIT7_Toggle=off
  MATLAB Function : MATLAB Function  TreatAsAtomicUnit=on  SystemSampleTime=T_s
  NOT : Logic  Operator=NOT  IconShape=distinctive  AllPortsSameDT=off  OutDataTypeStr=boolean
  Pulse Generator : DiscretePulseGenerator  Period=0.5/T_s  PulseWidth=0.25/T_s  SampleTime=T_s
  wires:
  Pulse Generator/1 -> MATLAB Function/3(blink)
  fault/1 -> MATLAB Function/2(fault)
  MATLAB Function/1(led) -> NOT/1
  reset/1 -> MATLAB Function/1(reset)
  enabled/1 -> Digital Output1/1
  NOT/1 -> Digital Output2/1

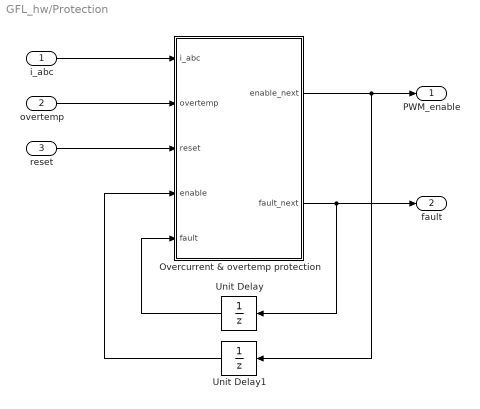
== system GFL_hw/Protection ==
  i_abc : Inport
  overtemp : Inport  Port=2
  reset : Inport  Port=3
  Overcurrent & overtemp protection : MATLAB Function  TreatAsAtomicUnit=on  SystemSampleTime=T_s
  Unit Delay : UnitDelay  InitialCondition=false  SampleTime=T_s  HasFrameUpgradeWarning=on
  Unit Delay1 : UnitDelay  InitialCondition=false  SampleTime=T_s  HasFrameUpgradeWarning=on
  PWM_enable : Outport
  fault : Outport  Port=2
  wires:
  i_abc/1 -> Overcurrent & overtemp protection/1(i_abc)
  overtemp/1 -> Overcurrent & overtemp protection/2(overtemp)
  reset/1 -> Overcurrent & overtemp protection/3(reset)
  Overcurrent & overtemp protection/1(enable_next) -> Unit Delay1/1, PWM_enable/1
  Overcurrent & overtemp protection/2(fault_next) -> Unit Delay/1, fault/1
  Unit Delay1/1 -> Overcurrent & overtemp protection/4(enable)
  Unit Delay/1 -> Overcurrent & overtemp protection/5(fault)

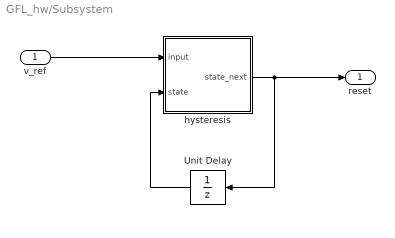
== system GFL_hw/Subsystem ==
  v_ref : Inport
  Unit Delay : UnitDelay  InitialCondition=false  SampleTime=T_s  HasFrameUpgradeWarning=on
  hysteresis : MATLAB Function  TreatAsAtomicUnit=on
  reset : Outport
  wires:
  v_ref/1 -> hysteresis/1(input)
  hysteresis/1(state_next) -> reset/1, Unit Delay/1
  Unit Delay/1 -> hysteresis/2(state)

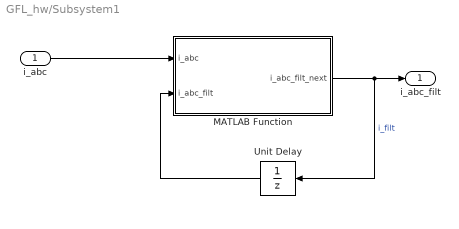
== system GFL_hw/Subsystem1 ==
  i_abc : Inport
  MATLAB Function : MATLAB Function  TreatAsAtomicUnit=on
  Unit Delay : UnitDelay  SampleTime=T_s  HasFrameUpgradeWarning=on
  i_abc_filt : Outport
  wires:
  MATLAB Function/1(i_abc_filt_next) -> Unit Delay/1, i_abc_filt/1  "i_filt"
  i_abc/1 -> MATLAB Function/1(i_abc)
  Unit Delay/1 -> MATLAB Function/2(i_abc_filt)

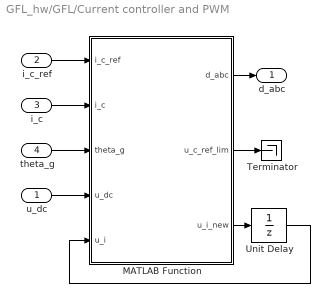
== system GFL_hw/GFL/Current controller and PWM ==
  u_dc : Inport
  i_c_ref : Inport  Port=2
  i_c : Inport  Port=3
  theta_g : Inport  Port=4
  MATLAB Function : MATLAB Function  TreatAsAtomicUnit=on
  Terminator : Terminator
  Unit Delay : UnitDelay  InitialCondition=u_gN  SampleTime=T_s  HasFrameUpgradeWarning=on
  d_abc : Outport  PortDimensions=3
  wires:
  MATLAB Function/3(u_i_new) -> Unit Delay/1
  i_c_ref/1 -> MATLAB Function/1(i_c_ref)
  i_c/1 -> MATLAB Function/2(i_c)
  Unit Delay/1 -> MATLAB Function/5(u_i)
  MATLAB Function/1(d_abc) -> d_abc/1
  theta_g/1 -> MATLAB Function/3(theta_g)
  u_dc/1 -> MATLAB Function/4(u_dc)
  MATLAB Function/2(u_c_ref_lim) -> Terminator/1

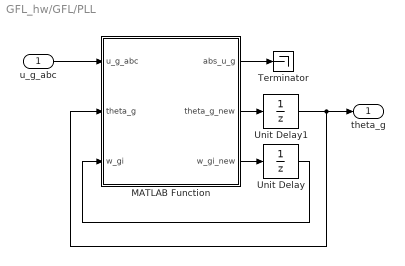
== system GFL_hw/GFL/PLL ==
  u_g_abc : Inport
  MATLAB Function : MATLAB Function  TreatAsAtomicUnit=on
  Terminator : Terminator
  Unit Delay : UnitDelay  InitialCondition=w_g  SampleTime=T_s  HasFrameUpgradeWarning=on
  Unit Delay1 : UnitDelay  SampleTime=T_s  HasFrameUpgradeWarning=on
  theta_g : Outport
  wires:
  u_g_abc/1 -> MATLAB Function/1(u_g_abc)
  MATLAB Function/3(w_gi_new) -> Unit Delay/1
  MATLAB Function/2(theta_g_new) -> Unit Delay1/1
  Unit Delay1/1 -> MATLAB Function/2(theta_g), theta_g/1
  Unit Delay/1 -> MATLAB Function/3(w_gi)
  MATLAB Function/1(abs_u_g) -> Terminator/1

== matlab function GFL_hw/Inputs & scaling/MATLAB Function8 ==
  data: adc input; y output
function y = fcn(adc)

y = (adc*80/4095-4.067)/1.0114 + 5;

== matlab function GFL_hw/Inputs & scaling/MATLAB Function10 ==
  data: adc input double; y output double
function y = fcn(adc)

ref_max = 1; % maximum desired value of the reference, i.e. the output will be 0...ref_max
y = max(0, ref_max*adc/4002);

== matlab function GFL_hw/Protection/Overcurrent & overtemp protection ==
  data: i_abc input double; enable_next output boolean; fault_next output boolean; overtemp input boolean; reset input boolean; enable input boolean; fault input boolean
function [enable_next, fault_next] = fcn(i_abc, overtemp, reset, enable, fault)

if(abs(i_abc(1))>=6 || abs(i_abc(2))>=6 || abs(i_abc(3))>=6)% || overtemp==true)
    fault_state=true;
else
    fault_state=false;
end

if(fault_state==true)
    fault_next=true;
    enable_next=false;
elseif(fault_state==false && reset==true)
    fault_next=false;
    enable_next=true;
else
    fault_next=fault;
    enable_next=enable;
end

== matlab function GFL_hw/LED control/MATLAB Function ==
  data: reset input boolean; led output; fault input boolean; blink input
function led = fcn(reset, fault, blink)

if(reset==true)
    led=1;
elseif(fault==true)
    led=blink;
else
    led=0;
end

== matlab function GFL_hw/Subsystem1/MATLAB Function ==
  data: i_abc input; i_abc_filt_next output; i_abc_filt input; w_g parameter; T_s parameter
function i_abc_filt_next = fcn(i_abc, i_abc_filt, w_g, T_s)

w_c=2*pi*w_g;
i_abc_filt_next =  i_abc_filt*(1 - w_c*T_s) + i_abc*(w_c*T_s);

== matlab function GFL_hw/GFL/Current controller and PWM/MATLAB Function ==
  settings: updateMethod=DISCRETE  sampleTime=T_s
  data: i_c_ref input size=1; i_c input size=1; theta_g input size=1; u_dc input size=1; u_i input size=1; w_g parameter size=1; L_f parameter size=1; alpha_c parameter size=1; T_s parameter size=1; d_abc output size=3; u_c_ref_lim output size=1; u_i_new output size=1
function [d_abc, u_c_ref_lim, u_i_new] = cc(i_c_ref, i_c, ...
    theta_g, u_dc, u_i, w_g, L_f, alpha_c, T_s)

%% Current controller 
% Gains
k_i = alpha_c^2*L_f;                % Integral gain
k_t = alpha_c*L_f;                  % Reference gain
k_p = (2*alpha_c - 1j*w_g)*L_f;     % Proportional gain

% Voltage reference in synchronous coordinates
u_c_ref = k_t*i_c_ref - k_p*i_c + u_i;

% Reference in stator coordinates
theta_gc = theta_g + 1.5*T_s*w_g;   % Compensation for discrete-time delays
u_cs_ref = u_c_ref*exp(1j*theta_gc);

%% Symmetrical suboscillation PWM
% Components of the voltage space vector
u_c_alpha_ref = real(u_cs_ref);
u_c_beta_ref  = imag(u_cs_ref);

% Phase-voltage references
u_ca_ref = u_c_alpha_ref;
u_cb_ref = .5*(-u_c_alpha_ref + sqrt(3)*u_c_beta_ref);
u_cc_ref = .5*(-u_c_alpha_ref - sqrt(3)*u_c_beta_ref);

% Vector of phase-voltage references
u_c_abc_ref = [u_ca_ref; u_cb_ref; u_cc_ref];

% Symmetrization of the references by adding the zero-sequence voltage
u0 = .5*(max(u_c_abc_ref) + min(u_c_abc_ref));
u_c_abc_ref = u_c_abc_ref - u0;

% Clipping of the reference voltages such that no phase error is caused. 
% If all phase voltage reference are realizable (below u_dc/2), m = 1 holds.
m = max([2*u_c_abc_ref/u_dc; 1]);
u_c_abc_ref = u_c_abc_ref/m;

% Duty cycles, which can be directly used for triangle comparison, 
% if the triangle wave varies between 0...1
d_abc = .5 + u_c_abc_ref/u_dc;

% Realized voltage vector is calculated from the clamped duty ratios.
% If the PWM does not saturate, u_c_ref_lim = u_c_ref holds. The realized
% voltage vector is needed, e.g., for the current-controller antiwindup.
u_cs_ref_lim = 2/3*(d_abc(1) + d_abc(2)*exp(1j*2*pi/3) ...
    + d_abc(3)*exp(1j*4*pi/3))*u_dc;
% In estimated rotor flux coordinates
u_c_ref_lim = exp(-1j*theta_gc)*u_cs_ref_lim;  

%% Update the integral state of the current controller 
u_i_new = u_i + T_s*k_i*(i_c_ref - i_c + (u_c_ref_lim - u_c_ref)/k_t);

== matlab function GFL_hw/GFL/Current reference ==
  settings: updateMethod=DISCRETE  sampleTime=T_s
  data: p_g_ref input; q_g_ref input; i_c_ref output; u_gN parameter size=1
function i_c_ref = curr_ref(p_g_ref, q_g_ref, u_gN)

% Current references in grid-voltage coordinates
i_cd_ref = (2*p_g_ref) / (3*u_gN);
i_cq_ref = (-2*q_g_ref) / (3*u_gN);

i_c_ref = i_cd_ref + 1j*i_cq_ref;

== matlab function GFL_hw/GFL/MATLAB Function ==
  settings: updateMethod=DISCRETE  sampleTime=T_s
  data: theta_g input size=1; i_c_abc input size=3; i_c output size=1
function i_c = abc2dq(theta_g, i_c_abc)

% Space-vector transformation
i_cs = 2/3*(i_c_abc(1) + i_c_abc(2)*exp(1j*2*pi/3) ...
    + i_c_abc(3)*exp(1j*4*pi/3));

% Coordinate transformation
i_c = i_cs*exp(-1j*theta_g);

== matlab function GFL_hw/GFL/PLL/MATLAB Function ==
  settings: updateMethod=DISCRETE  sampleTime=T_s
  data: u_g_abc input size=3; theta_g input; w_gi input; u_gN parameter; w0_pll parameter; abs_u_g output size=1; theta_g_new output; w_gi_new output; T_s parameter
function [abs_u_g, theta_g_new, w_gi_new] = pll(u_g_abc, ...
    theta_g, w_gi, u_gN, w0_pll, T_s)

% Parameters 
% (Tuning of the PLL is analogous to that of the DC-voltage controller.)
zeta = 1;   % Damping ratio
k_p = 2*zeta*w0_pll/u_gN; 
k_i = w0_pll^2/u_gN;

% Space-vector transformation from phase-to-neutral components
u_gs = 2/3*(u_g_abc(1) + u_g_abc(2)*exp(1j*2*pi/3) + u_g_abc(3)*exp(1j*4*pi/3));

% Coordinate transformation to the "estimated" grid coordinates
u_g = exp(-1j*theta_g)*u_gs;

% Error signal, which is drive to zero by the PLL
u_gq = imag(u_g);

w_g = k_p*u_gq + w_gi;

% Update the integral state
w_gi_new = w_gi + T_s*k_i*u_gq;

% Update the grid-voltage angle
theta_g_new = theta_g + T_s*w_g;
while(theta_g_new > pi)
    theta_g_new = theta_g_new - 2*pi;
end
while(theta_g_new < -pi)
    theta_g_new = theta_g_new + 2*pi;
end

% Absolute value of the grid-voltage vector
abs_u_g = abs(u_g);

== matlab function GFL_hw/Inputs & scaling/MATLAB Function1 ==
  data: i_adc input; i_real output
function i_real = fcn(i_adc)

i_real = -0.0075*i_adc + 15.4645;

== matlab function GFL_hw/Inputs & scaling/MATLAB Function ==
  data: i_adc input; i_real output
function i_real = fcn(i_adc)

i_real = -0.0075*i_adc + 15.4645;

== matlab function GFL_hw/Inputs & scaling/MATLAB Function2 ==
  data: i_adc input; i_real output
function i_real = fcn(i_adc)

i_real = -0.0075*i_adc + 15.4645;

== matlab function GFL_hw/Subsystem/hysteresis ==
  data: input input; state input; state_next output
function state_next = fcn(input, state)

if(state==false && input>=0.9)
    state_next=true;
elseif(state==true && input<=0.1)
    state_next=false;
else
    state_next=state;
end

== matlab function GFL_hw/Inputs & scaling/MATLAB Function9 ==
  data: adc input; y output
function y = fcn(adc)

y = (adc*80/4095-4.067)/1.0114 + 5;

== matlab function GFL_hw/Inputs & scaling/MATLAB Function4 ==
  data: adc input; y output
function y = fcn(adc)

y = (adc*80/4095-4.067)/1.0114 + 5;

== matlab function GFL_hw/Inputs & scaling/MATLAB Function3 ==
  data: adc input; y output
function y = fcn(adc)

y = (adc*80/4095-4.067)/1.0114 + 5;

== matlab function GFL_hw/Inputs & scaling/MATLAB Function5 ==
  data: adc input; y output
function y = fcn(adc)

y = (adc*80/4095-4.067)/1.0114 + 5;

== matlab function GFL_hw/Inputs & scaling/MATLAB Function6 ==
  data: adc input; y output
function y = fcn(adc)

y = (adc*80/4095-4.067)/1.0114 + 5;

== matlab function GFL_hw/Inputs & scaling/MATLAB Function7 ==
  data: adc input; y output
function y = fcn(adc)

y = (adc*80/4095-4.067)/1.0114 + 5;
